simulink model "mqtt_send_func"  (R2022b)
settings: Solver=VariableStepAuto  StartTime=0.0  StopTime=10.0  RelTol=1e-3
settings Model: Creator=rishi  LastModifiedBy=rishi

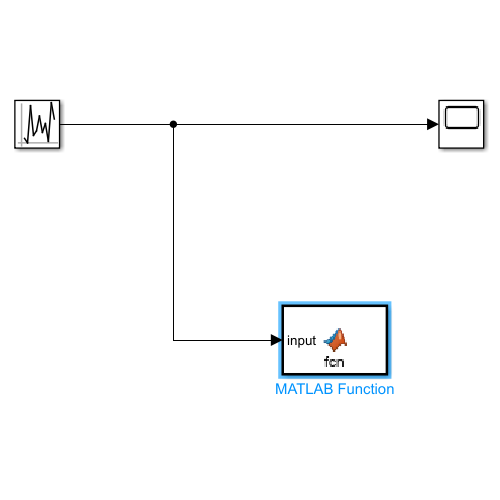
[thumbnail: Simulink's stored preview of the top-level diagram]
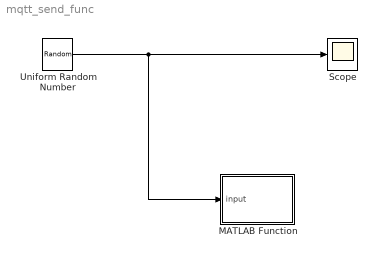
== system mqtt_send_func ==
  MATLAB Function : MATLAB Function  TreatAsAtomicUnit=on
  Scope : Scope
  Uniform Random Number : UniformRandomNumber  SampleTime=0.1
  wires:
  Uniform Random Number/1 -> Scope/1, MATLAB Function/1(input)

== matlab function mqtt_send_func/MATLAB Function ==
  data: input input
function fcn(input)
    %% Global variables
    BROKER_IP='192.168.1.74'; % IP of the Mosquitto broker
    BROKER_PORT=1883;         % default port 
    CLIENT_ID="matlabclient";% client ID
    KEEP_ALIVE=60;            % Keepalive timer
    PROTO="tcp";              % Transport Protocol
    TOPIC="test/matlab";       % topic 

    client=mqttclient(PROTO+"://"+BROKER_IP, ...
                  'Port',BROKER_PORT, ...
                  "ClientID",CLIENT_ID, ...
                  "KeepAliveDuration",KEEP_ALIVE);

    message=input;
    write(client,TOPIC,message);
